simulink model "ROS_test"  (R2017b)
settings: Solver=FixedStepAuto  StartTime=0.0  StopTime=50  FixedStep=0.01  RelTol=1e-3
undefined symbols (not defined in the file or in its folder): Angular, Linear
libraries: robotlib x3, simulink x3
settings Model: Creator=songkai  LastModifiedBy=songkai

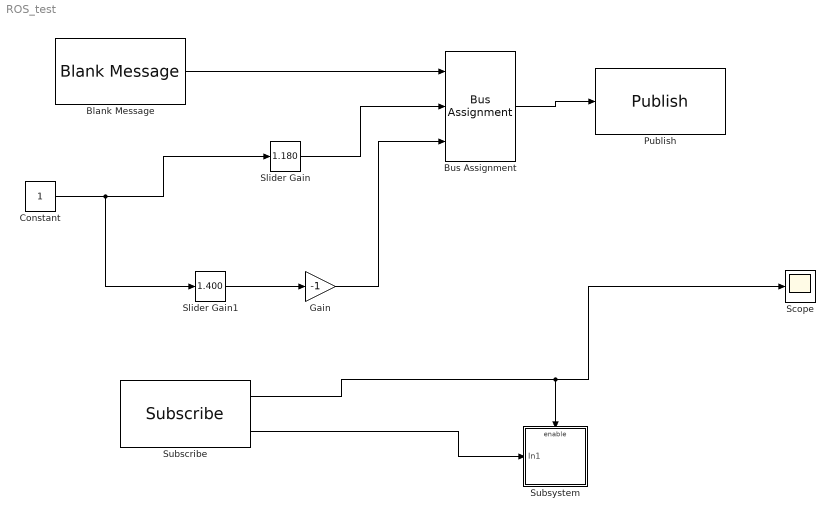
== system ROS_test ==
  Blank Message : robotlib/Blank Message  SourceLibraryInfo=This block requires Robotics System Toolbox  messageType=geometry_msgs/Twist  SampleTime=0.01
      settings: SourceProductBaseCode=RO
  Bus Assignment : BusAssignment  AssignedSignals=Linear.X,Angular.Z
  Constant : Constant
  Gain : Gain  Gain=-1
  Publish : robotlib/Publish  SourceLibraryInfo=This block requires Robotics System Toolbox  topicSource=Select from ROS network  topic=/mobile_base/commands/velocity  messageType=geometry_msgs/Twist  messageQueueLength=1
      link override SinkBlock: ROSTopic=/mobile_base/commands/velocity  ROSMessageType=geometry_msgs/Twist  SLBusName=SL_Bus_ROS_test_geometry_msgs_Twist  ModelName=ROS_test  BlockId=Pub_ROS_test_22
      settings: SourceProductBaseCode=RO
  Scope : Scope
  Slider Gain : simulink/Math Operations/Slider Gain  gain=1.180  low=0  high=2
  Slider Gain1 : simulink/Math Operations/Slider Gain  gain=1.400  low=-1  high=4
  Subscribe : robotlib/Subscribe  SourceLibraryInfo=This block requires Robotics System Toolbox  topicSource=Select from ROS network  topic=/odom  messageType=nav_msgs/Odometry  sampleTime=-1  messageQueueLength=1
      settings: SourceProductBaseCode=RO
  Subsystem : Subsystem
  wires:
  Bus Assignment/1 -> Publish/1
  Blank Message/1 -> Bus Assignment/1
  Constant/1 -> Slider Gain1/1, Slider Gain/1
  Subscribe/2 -> Subsystem/1(In1)
  Subscribe/1 -> Scope/1, Subsystem/Enable
  Slider Gain/1 -> Bus Assignment/2
  Slider Gain1/1 -> Gain/1
  Gain/1 -> Bus Assignment/3

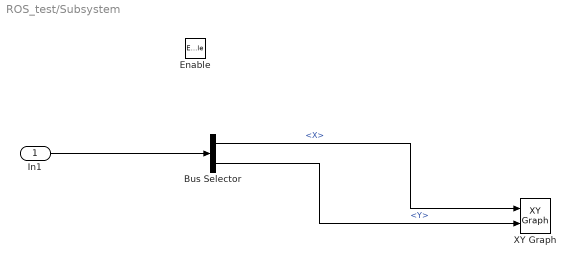
== system ROS_test/Subsystem ==
  In1 : Inport
  Enable : EnablePort
  Bus Selector : BusSelector  OutputSignals=Pose.Pose.Position.X,Pose.Pose.Position.Y
  XY Graph : simulink/Sinks/XY Graph  xmin=-50  xmax=50  ymin=-50  ymax=50  st=-1
  wires:
  Bus Selector/1 -> XY Graph/1  "<X>"
  Bus Selector/2 -> XY Graph/2  "<Y>"
  In1/1 -> Bus Selector/1
